simulink model "simpleBEV"  (R2018a)
settings: Solver=VariableStepAuto  StartTime=0.0  StopTime=600  RelTol=1e-3
libraries: autolibshared x1
settings Model: Creator=carca  LastModifiedBy=carca

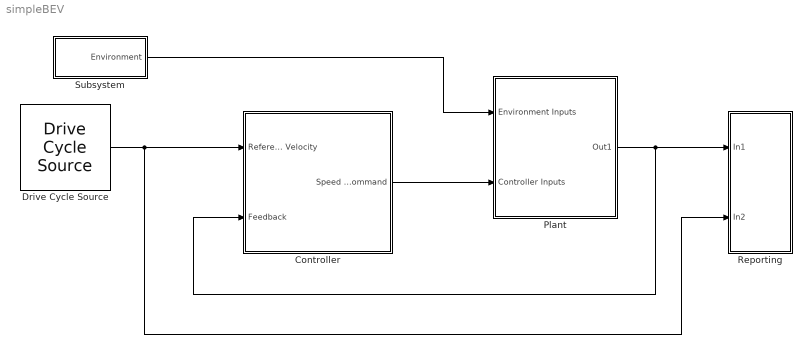
== system simpleBEV ==
  Controller : Subsystem
  Drive Cycle Source : autolibshared/Drive Cycle Source  cycleVar=US06  fileVar=cycleFTP75.mat  tfinal="600  seconds"  cycleRepeat=off  outAccPort=off  outGearPort=off  gearList=No gear data  t_wot1=5  xdot_woto=0  xdot_wot1=30  t_wot2=20  xdot_wot2=0  t_wotend=30  srcUnit=m/s  outUnit=m/s  srcAccUnit=m/s/s  outAccUnit=m/s^2  dt=0  aMode=1
      settings: SourceProductName=Powertrain Blockset  SourceProductBaseCode=PW
  Plant : Subsystem
  Reporting : Subsystem
  Subsystem : Subsystem
  wires:
  Drive Cycle Source/1 -> Reporting/2(In2), Controller/1(Reference Velocity)
  Controller/1(Speed Command) -> Plant/2(Controller Inputs)
  Plant/1(Out1) -> Controller/2(Feedback), Reporting/1(In1)
  Subsystem/1(Environment) -> Plant/1(Environment Inputs)

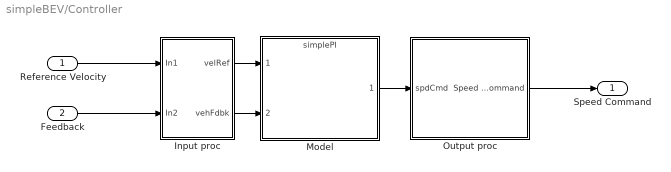
== system simpleBEV/Controller ==
  Reference Velocity : Inport
  Feedback : Inport  Port=2
  Input proc : Subsystem
  Model : ModelReference  ModelNameDialog=simplePI.slx  SimulationMode=Normal  ModelReferenceVersion=1.1
  Output proc : Subsystem
  Speed Command : Outport
  wires:
  Reference Velocity/1 -> Input proc/1(In1)
  Feedback/1 -> Input proc/2(In2)
  Output proc/1(Speed Command) -> Speed Command/1
  Input proc/2(vehFdbk) -> Model/2
  Input proc/1(velRef) -> Model/1
  Model/1 -> Output proc/1(spdCmd)

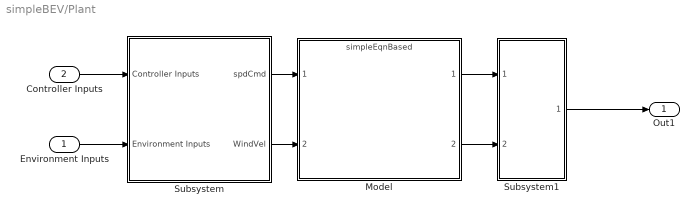
== system simpleBEV/Plant ==
  Environment Inputs : Inport
  Controller Inputs : Inport  Port=2
  Model : ModelReference  ModelNameDialog=simpleEqnBased.slx  SimulationMode=Normal  ModelReferenceVersion=1.4
  Subsystem : Subsystem
  Subsystem1 : Subsystem
  Out1 : Outport
  wires:
  Subsystem1/1(VehFdbk) -> Out1/1
  Controller Inputs/1 -> Subsystem/1(Controller Inputs)
  Environment Inputs/1 -> Subsystem/2(Environment Inputs)
  Subsystem/2(WindVel) -> Model/2
  Subsystem/1(spdCmd) -> Model/1
  Model/1 -> Subsystem1/1(VehSpd)
  Model/2 -> Subsystem1/2(WhlSlip)

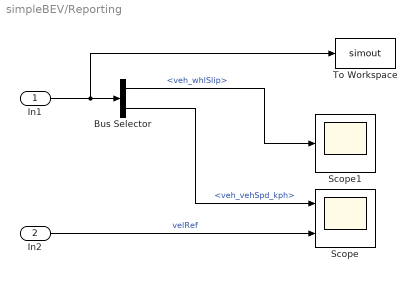
== system simpleBEV/Reporting ==
  In1 : Inport
  In2 : Inport  Port=2
  Bus Selector : BusSelector  OutputSignals=veh_whlSlip,veh_vehSpd_kph
  Scope : Scope  NumInputPorts=2
  Scope1 : Scope
  To Workspace : ToWorkspace  VariableName=simout  SaveFormat=Timeseries  SampleTime=-1
  wires:
  In1/1 -> Bus Selector/1, To Workspace/1
  Bus Selector/1 -> Scope1/1  "<veh_whlSlip>"
  Bus Selector/2 -> Scope/1  "<veh_vehSpd_kph>"
  In2/1 -> Scope/2  "velRef"

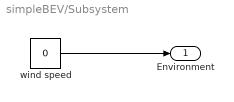
== system simpleBEV/Subsystem ==
  wind speed : Constant  Value=0
  Environment : Outport
  wires:
  wind speed/1 -> Environment/1

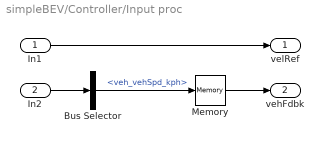
== system simpleBEV/Controller/Input proc ==
  In1 : Inport
  In2 : Inport  Port=2
  Bus Selector : BusSelector  OutputSignals=veh_vehSpd_kph
  Memory : Memory
  velRef : Outport
  vehFdbk : Outport  Port=2
  wires:
  In1/1 -> velRef/1
  In2/1 -> Bus Selector/1
  Bus Selector/1 -> Memory/1  "<veh_vehSpd_kph>"
  Memory/1 -> vehFdbk/1

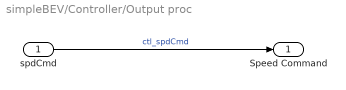
== system simpleBEV/Controller/Output proc ==
  spdCmd : Inport
  Speed Command : Outport
  wires:
  spdCmd/1 -> Speed Command/1  "ctl_spdCmd"

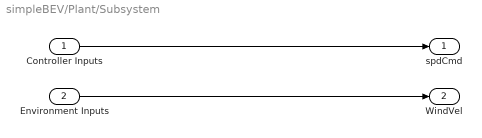
== system simpleBEV/Plant/Subsystem ==
  Controller Inputs : Inport
  Environment Inputs : Inport  Port=2
  spdCmd : Outport
  WindVel : Outport  Port=2
  wires:
  Environment Inputs/1 -> WindVel/1
  Controller Inputs/1 -> spdCmd/1

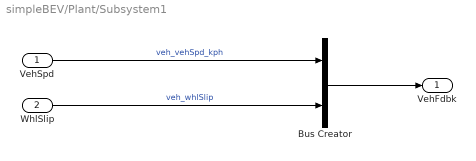
== system simpleBEV/Plant/Subsystem1 ==
  VehSpd : Inport
  WhlSlip : Inport  Port=2
  Bus Creator : BusCreator  Inputs=2
  VehFdbk : Outport
  wires:
  VehSpd/1 -> Bus Creator/1  "veh_vehSpd_kph"
  Bus Creator/1 -> VehFdbk/1
  WhlSlip/1 -> Bus Creator/2  "veh_whlSlip"
